simulink model "pendulum_3a"  (R2018a)
settings: Solver=VariableStepAuto  StartTime=0.0  StopTime=30.0  RelTol=1e-3
values from neighbouring files (symbols this model uses):
  A = [0 0 1 0;0 0 0 1;0 -Rod_m*g/Cart_m -(Kg^2)*Km*Kb/(Cart_m*Rm*motor_radius^2) 0 ... (first row only)    [pendulum_version1.m]
  B = [0;0;Km*Kg/(Cart_m*Rm*motor_radius);-Km*Kg/(Cart_m*Rm*motor_radius*Rod_l)]    [pendulum_version1.m]
  C = [1 0 0 0 ... (first row only)    [pendulum_version1.m]
  CC = eye(n_outputs)    [pendulum_version1.m]
  K = lqr(A,B,Q,R)    [pendulum_version1.m]
  Ts = 1/200    (= 0.005)    [pendulum_version1.m]
  xd = 1    [pendulum_version1.m]
undefined symbols (not defined in the file or in its folder): omega_c
settings Model: Creator=paul-emileverleye  LastModifiedBy=paul-emileverleye

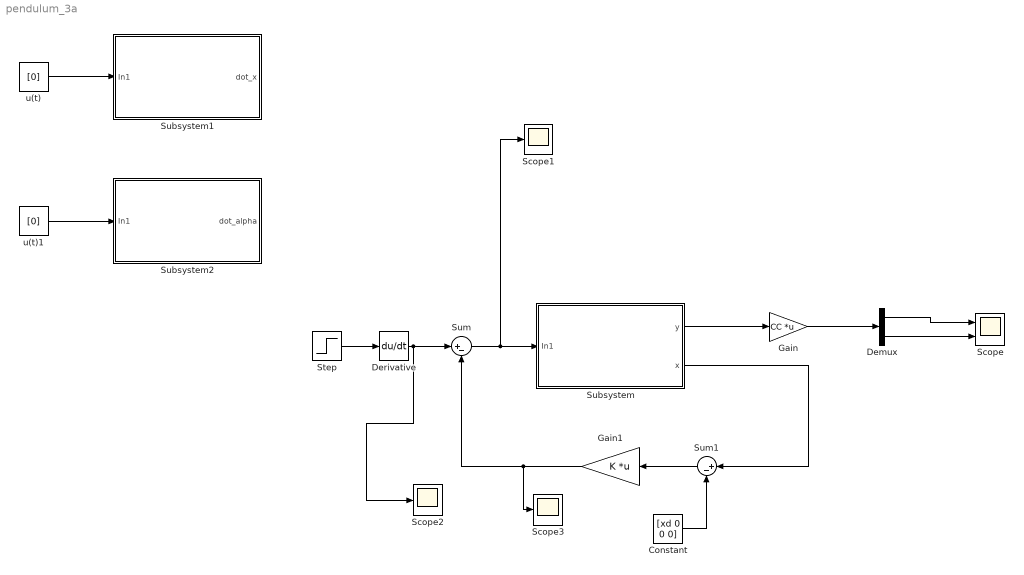
== system pendulum_3a ==
  Constant : Constant  Value=[xd 0 0 0]
  Demux : Demux  Outputs=2
  Derivative : Derivative
  Gain : Gain  Gain=CC  Multiplication=Matrix(K*u)
  Gain1 : Gain  Gain=K  Multiplication=Matrix(K*u)
  Scope : Scope  NumInputPorts=2
  Scope1 : Scope
  Scope2 : Scope
  Scope3 : Scope
  Step : Step  SampleTime=0
  Subsystem : Subsystem
  Subsystem1 : Subsystem
  Subsystem2 : Subsystem
  Sum : Sum  Inputs=|+-
  Sum1 : Sum  Inputs=|+-
  u(t) : Constant  Value=[0]
  u(t)1 : Constant  Value=[0]
  wires:
  Gain1/1 -> Scope3/1, Sum/2
  Sum/1 -> Subsystem/1(In1), Scope1/1
  Demux/1 -> Scope/1
  Gain/1 -> Demux/1
  Demux/2 -> Scope/2
  Subsystem/1(y) -> Gain/1
  Sum1/1 -> Gain1/1
  Constant/1 -> Sum1/2
  Step/1 -> Derivative/1
  Derivative/1 -> Scope2/1, Sum/1
  Subsystem/2("x ") -> Sum1/1
  u(t)/1 -> Subsystem1/1(In1)
  u(t)1/1 -> Subsystem2/1(In1)

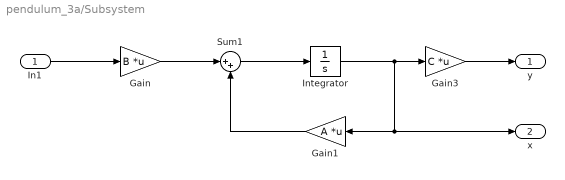
== system pendulum_3a/Subsystem ==
  In1 : Inport
  Gain : Gain  Gain=B  Multiplication=Matrix(K*u)
  Gain1 : Gain  Gain=A  Multiplication=Matrix(K*u)
  Gain3 : Gain  Gain=C  Multiplication=Matrix(K*u)
  Integrator : Integrator
  Sum1 : Sum  Inputs=|++
  y : Outport
  "x " : Outport  Port=2
  wires:
  In1/1 -> Gain/1
  Gain/1 -> Sum1/1
  Sum1/1 -> Integrator/1
  Integrator/1 -> Gain3/1, "x "/1, Gain1/1
  Gain1/1 -> Sum1/2
  Gain3/1 -> y/1

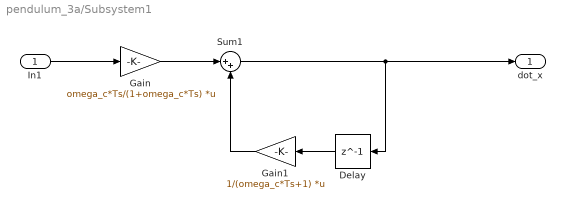
== system pendulum_3a/Subsystem1 ==
  In1 : Inport
  Delay : Delay  DelayLength=1  InitialCondition=0
  Gain : Gain  Gain=omega_c*Ts/(1+omega_c*Ts)  Multiplication=Matrix(K*u)
  Gain1 : Gain  Gain=1/(omega_c*Ts+1)  Multiplication=Matrix(K*u)
  Sum1 : Sum  Inputs=|++
  dot_x : Outport
  wires:
  In1/1 -> Gain/1
  Gain/1 -> Sum1/1
  Sum1/1 -> Delay/1, dot_x/1
  Delay/1 -> Gain1/1
  Gain1/1 -> Sum1/2

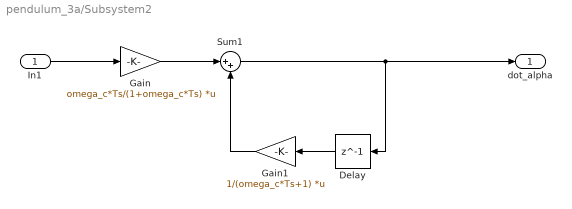
== system pendulum_3a/Subsystem2 ==
  In1 : Inport
  Delay : Delay  DelayLength=1  InitialCondition=0
  Gain : Gain  Gain=omega_c*Ts/(1+omega_c*Ts)  Multiplication=Matrix(K*u)
  Gain1 : Gain  Gain=1/(omega_c*Ts+1)  Multiplication=Matrix(K*u)
  Sum1 : Sum  Inputs=|++
  "dot_alpha " : Outport
  wires:
  In1/1 -> Gain/1
  Gain/1 -> Sum1/1
  Sum1/1 -> Delay/1, "dot_alpha "/1
  Delay/1 -> Gain1/1
  Gain1/1 -> Sum1/2
